simulink model "ZeroCrossing"  (R2022b)
settings: Solver=FixedStepDiscrete  StartTime=0.0  StopTime=20  FixedStep=1e-3  RelTol=1e-3
settings Model: Creator=ahmed  LastModifiedBy=ahmed

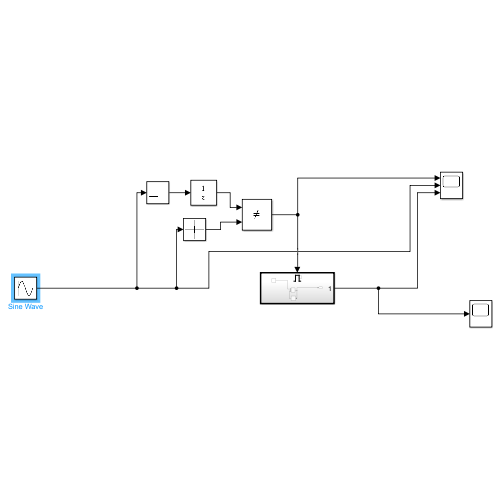
[thumbnail: Simulink's stored preview of the top-level diagram]
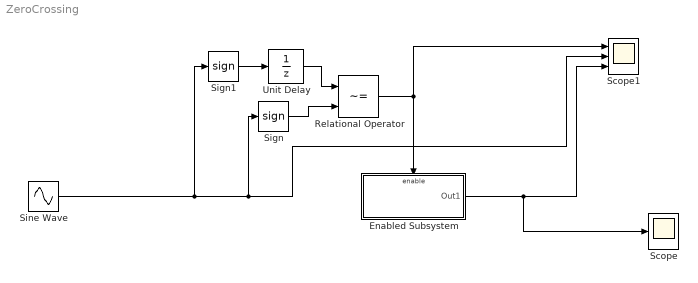
== system ZeroCrossing ==
  Enabled Subsystem : Subsystem  TreatAsAtomicUnit=on
  Relational Operator : RelationalOperator  Operator=~=  OutDataTypeStr=boolean  RndMeth=Simplest  InputSameDT=off
  Scope : Scope
  Scope1 : Scope  NumInputPorts=3
  Sign : Signum
  Sign1 : Signum
  Sine Wave : Sin  Frequency=2  SampleTime=0
  Unit Delay : UnitDelay  SampleTime=-1  HasFrameUpgradeWarning=on
  wires:
  Sine Wave/1 -> Sign1/1, Sign/1, Scope1/2
  Enabled Subsystem/1(Out1) -> Scope/1, Scope1/3
  Relational Operator/1 -> Scope1/1, Enabled Subsystem/Enable
  Sign/1 -> Relational Operator/2
  Sign1/1 -> Unit Delay/1
  Unit Delay/1 -> Relational Operator/1

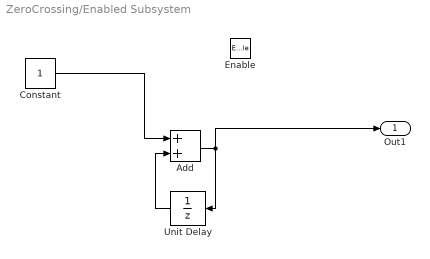
== system ZeroCrossing/Enabled Subsystem ==
  Enable : EnablePort
  Add : Sum
  Constant : Constant
  Unit Delay : UnitDelay  SampleTime=-1  HasFrameUpgradeWarning=on
  Out1 : Outport
  wires:
  Constant/1 -> Add/1
  Add/1 -> Unit Delay/1, Out1/1
  Unit Delay/1 -> Add/2
